simulink model "ClosedLoopControl"  (R2016b)
settings: Solver=FixedStepDiscrete  StartTime=0.0  StopTime=Inf  FixedStep=sCoreParams.core.stepPeriod  RelTol=1e-3  EnableMultiTasking=on
undefined symbols (not defined in the file): fdesignblkfcn, gcbh, High, sCoreParams, sCoreParams_decoders_chanceDetector_randStimEventsPerSec, sCoreParams_decoders_txDetector_channel1, sCoreParams_decoders_txDetector_channel2, sCoreParams_decoders_txDetector_detectChannelInds, sCoreParams_decoders_txDetector_nChannels, sCoreParams_Features_Baseline_initialThresholdValue, sCoreParams_Features_Baseline_weightPreviousThreshold, sCoreParams_Features_Data_SmoothWindowsDurationSamples, sCoreParams_stimulator_stimAfterDelaySteps
libraries: dsparch4 x20, dspstat3 x19, dspspect3 x6, dspfdesign x2, dspindex x2, dspswit3 x1
(part 6 of 6)

== system ClosedLoopControl/FilterBanks/Variant FILTER 2000/65-200Hz HighGammaRipple FIR ==
  EEGData : Inport
  Generated Filter Block : DiscreteFir  Tag=BlockMethodSubSystem  Coefficients=[0.043674950645707943 -0.010510801076776438 -0.0092198604406533054 -0.0078072197440863019 -0.0061576291109547441 -0.0043314949479796505 -0.0026149837714866844 -0.0014281197315007387 -0.0011887830977032846 -0.0020631394359844836 -0.0038906609829976006 -0.006134979543899413 -0.0080743521554436769 -0.0090186910392010006 -0.0085928718984132329 -0.0068824719973744029 -0.0044344002598706734 -0.0020632098371482117 -0.00054620058864337216 -0.00031706926836648172 -0.0012806039208504247 -0.0028303540771732584 -0.0040768356042938676 -0.004193132697654047 -0.0027660676413756961 1.9003693936618729e-05 0.0034067519279456487 0.0063472526354222602 0.0078958974614977504 0.0075793823939889725 0.0056281036442865778 0.0028514070097576216 0.00042987516134896416 -0.00071303834093239911 1.1697363323633972e-05 0.0020369008242335485 0.0045707172575817877 0.0063400232285504843 0.006152335767163339 0.003695198751154251 -0.00054923784249524951 -0.0052930021300986009 -0.009082894815013105 -0.010679189468049901 -0.009713948692912408 -0.0067468353855187129 -0.0031802128714443988 -0.00063228620545409213 -0.00035139072256231481 -0.0026086409852362456 -0.0065830274486462651 -0.010571501918713583 -0.012689614383126465 -0.011577477565379819 -0.0070576745373317736 -0.00022999532853976319 0.0068154951113979841 0.011843234875324286 0.013289460151243533 0.011001391875699177 0.0063095176650106582 0.0016313362199767314 -0.00052119400123590027 0.0014569178651438908 0.0074726777669980133 0.015628713969671838 0.022826703629726497 0.025893486581749524 0.022907578453487763 0.014019972540609493 0.0016645482174998925 -0.010167457554019462 -0.017562158381230882 -0.0180477323755667 -0.01194498020464765 -0.0024264873025872094 0.0052207045747070255 0.0056493327084122186 -0.0045373885153166225 -0.025015012812241458 -0.051246002878708945 -0.075349015080128312 -0.088355355358379697 -0.083035398155685114 -0.056553784398185536 -0.011862247095400281 0.042515847778265718 0.094576601537287724 0.13197925194672577 0.14558091380700244 0.13197925194672577 0.094576601537287724 0.042515847778265718 -0.011862247095400281 -0.056553784398185536 -0.083035398155685114 -0.088355355358379697 -0.075349015080128312 -0.051246002878708945 -0.025015012812241458 -0.0045373885153166225 0.0056493327084122186 0.0052207045747070255 -0.0024264873025872094 -0.01194498020464765 -0.0180477323755667 -0.017562158381230882 -0.010167457554019462 0.0016645482174998925 0.014019972540609493 0.022907578453487763 0.025893486581749524 0.022826703629726497 0.015628713969671838 0.0074726777669980133 0.0014569178651438908 -0.00052119400123590027 0.0016313362199767314 0.0063095176650106582 0.011001391875699177 0.013289460151243533 0.011843234875324286 0.0068154951113979841 -0.00022999532853976319 -0.0070576745373317736 -0.011577477565379819 -0.012689614383126465 -0.010571501918713583 -0.0065830274486462651 -0.0026086409852362456 -0.00035139072256231481 -0.00063228620545409213 -0.0031802128714443988 -0.0067468353855187129 -0.009713948692912408 -0.010679189468049901 -0.009082894815013105 -0.0052930021300986009 -0.00054923784249524951 0.003695198751154251 0.006152335767163339 0.0063400232285504843 0.0045707172575817877 0.0020369008242335485 1.1697363323633972e-05 -0.00071303834093239911 0.00042987516134896416 0.0028514070097576216 0.0056281036442865778 0.0075793823939889725 0.0078958974614977504 0.0063472526354222602 0.0034067519279456487 1.9003693936618729e-05 -0.0027660676413756961 -0.004193132697654047 -0.0040768356042938676 -0.0028303540771732584 -0.0012806039208504247 -0.00031706926836648172 -0.00054620058864337216 -0.0020632098371482117 -0.0044344002598706734 -0.0068824719973744029 -0.0085928718984132329 -0.0090186910392010006 -0.0080743521554436769 -0.006134979543899413 -0.0038906609829976006 -0.0020631394359844836 -0.0011887830977032846 -0.0014281197315007387 -0.0026149837714866844 -0.0043314949479796505 -0.0061576291109547441 -0.0078072197440863019 -0.0092198604406533054 -0.010510801076776438 0.043674950645707943]  InputProcessing=Columns as channels (frame based)
  filteredData : Outport
  wires:
  EEGData/1 -> Generated Filter Block/1
  Generated Filter Block/1 -> filteredData/1

== system ClosedLoopControl/FilterBanks/Variant FILTER 2000/65-200Hz HighGammaRipple IIR ==
  EEGData : Inport
  Generated Filter Block : dsparch4/Biquad Filter  Tag=BlockMethodSubSystem  IIRFiltStruct=Direct form II  CoeffSource=Specify via dialog  BiQuadCoeffs=[0.67667743659925317 0 -0.67667743659925317 1 -1.791106372362715 0.84351743161553339;0.20837637004489881 0 -0.20837637004489881 1 -1.4769568640840638 0.82858480682365565;0.21913950715217931 0 -0.21913950715217931 1 -1.3946221573759421 0.62632638513627259;0.13404107548876229 0 -0.13404107548876229 1 -1.4634270346154397 0.61227676045926838;0.22926259000998553 0 -0.22926259000998553 1 -1.4248965089945402 0.73918023284028478;0.1662719018063869 0 -0.1662719018063869 1 -1.6043511746437273 0.69199629969542564;0.071396379929834025 0 -0.071396379929834025 1 -1.9317179351880835 0.97744998664625005;0.26148164315809597 0 -0.26148164315809597 1 -1.5540993535626753 0.93822820155749087;0.25565951467668901 0 -0.25565951467668901 1 -1.7364105251114004 0.79566729073556186;0.21891419381257862 0 -0.21891419381257862 1 -1.6744829666918539 0.74473352537242943;0.16735244352374978 0 -0.16735244352374978 1 -1.4166978728907922 0.60600668409114;0.2415146980022162 0 -0.2415146980022162 1 -1.3974831127623975 0.6713282499392339;0.26540418737962024 0 -0.26540418737962024 1 -1.5300311665420243 0.64388417032152689;0.10300734712666591 0 -0.10300734712666591 1 -1.8869858981947756 0.93319650449939318;2 0 -2 1 -1.8406560359772179 0.88897180839051049]  a0Flag=Warning  IC=0  ICnum=0  ICden=0  InputProcessing=Columns as channels (frame based)  denAccumFracLength=30  denProdOutputFracLength=30  secondMemoryFracLength=15  roundingMode=Floor  overflowMode=off  ScaleValues=[0.034709882337591945;1;1;1;1;1;1;1;1;1;1;1;1;1;1;1.0919362488362816]  optimizeScaleValues=off  ScaleValueMode=Specify via input port (g)  scaleValueFracLength=14  FilterSource=Specify via dialog  FilterObject=BQF
  filteredData : Outport
  wires:
  EEGData/1 -> Generated Filter Block/1
  Generated Filter Block/1 -> filteredData/1

== system ClosedLoopControl/FilterBanks/Variant FILTER 2000/8-15Hz Alpha FIR ==
  EEGData : Inport
  Generated Filter Block : DiscreteFir  Tag=BlockMethodSubSystem  Coefficients=[1.1166843982614926e-06 -5.1505963497875887e-06 -1.2812602333555129e-05 -2.1871054990882468e-05 -3.2323373818540652e-05 -4.4162634838047868e-05 -5.7377540676991869e-05 -7.195240245586386e-05 -8.7867133639842035e-05 -0.00010509725598372113 -0.00012361391766630315 -0.00014338392367813367 -0.000164369778493665 -0.00018652974102566303 -0.00020981789182618625 -0.0002341842124648283 -0.0002595746769810637 -0.00028593135527383055 -0.00031319252825774447 -0.00034129281458180586 -0.00037016330867327857 -0.00039973172983648352 -0.00042992258210380332 -0.00046065732450443646 -0.00049185455138502153 -0.00052343018238589314 -0.000555297661646971 -0.0005873681657885076 -0.00061955082018408858 -0.00065175292301663287 -0.00068388017658249981 -0.00071583692528446631 -0.00074752639973140443 -0.00077885096634068161 -0.00080971238181931681 -0.00084001205188102607 -0.00086965129353934944 -0.00089853160030159028 -0.0009265549095744043 -0.00095362387157998788 -0.00097964211907159478 -0.0010045145371285577 -0.0010281475323047058 -0.0010504493003992363 -0.0010713300921165658 -0.0010907024758808866 -0.0011084815970723843 -0.0011245854329553625 -0.00113893504257369 -0.0011514548108961891 -0.001162072686503848 -0.0011707204121218695 -0.0011773337473127315 -0.0011818526826615754 -0.0011842216448022078 -0.0011843896916509528 -0.0011823106972363748 -0.0011779435255354414 -0.00117125219275111 -0.0011622060174923557 -0.0011507797583454361 -0.001136953738354511 -0.0011207139559606311 -0.0011020521819804436 -0.0010809660422397137 -0.001057459085511797 -0.0010315408364474827 -0.0010032268332200427 -0.00097253864964778316 -0.00093950390159584351 -0.00090415623749921738 -0.00086653531289007147 -0.00082668674885407638 -0.00078466207438273922 -0.00074051865263137029 -0.00069431959113537079 -0.0006461336360806941 -0.00059603505076769926 -0.00054410347845094465 -0.00049042378978056769 -0.0004350859151140158 -0.00037818466200922462 -0.0003198195182527428 -0.00026009444081761201 -0.00019911763118664756 -0.00013700129751690498 -7.3861404160011573e-05 -9.8174090911267554e-06 5.5008010163797022e-05 0.00012048924147724876 0.00018649803328639865 0.00025290379928409514 0.00031957393191114501 0.00038637412389685354 0.00045316869706702476 0.00051982093761261162 0.00058619343698820684 0.00065214843758748075 0.00071754818232275524 0.00078225526721801533 0.00084613299610908864 0.00090904573653135254 0.00097085927586427958 0.0010314411767934721 0.0010906611311446244 0.0011483913111399052 0.0012045067171260633 0.0012588855208245753 0.0013114094031579228 0.0013619638857121615 0.0014104386549047448 0.0014567278779377545 0.0015007305096304167 0.0015423505892410412 0.0015814975264072709 0.001618086375354588 0.0016520380965466808 0.0016832798049771526 0.0017117450043303123 0.0017373738062692796 0.0017601131341423238 0.0017799169104332252 0.0017967462273182613 0.0018105694997313348 0.0018213626003794627 0.0018291089761933916 0.0018337997457423454 0.0018354337771877447 0.0018340177463980255 0.0018295661748954481 0.0018221014473556757 0.0018116538084320456 0.0017982613387285684 0.0017819699097986867 0.0017628331181006056 0.0017409121978943678 0.0017162759131207782 0.0016890004283574528 0.0016591691590027344 0.0016268726008937253 0.001592208139620101 0.0015552798398505627 0.0015161982150436648 0.0014750799779690521 0.0014320477725188181 0.0013872298873415828 0.0013407599518838245 0.0012927766154738488 0.001243423210133381 0.0011928473978500983 0.0011412008030911467 0.0010886386313827949 0.0010353192748249133 0.00098140390545031655 0.0009270560573785804 0.00087244119875139019 0.00081772629447154682 0.00076307936080061199 0.00070866901290059193 0.00065466400643282975 0.00060123277435255879 0.00054854296006001896 0.00049676094808876381 0.00044605139352870261 0.00039657675139517979 0.00034849680716653192 0.0003019682097202846 0.00025714400790310016 0.00021417319197122785 0.00017320024113676101 0.00013436467845048239 9.7800634244212941e-05 6.3636419344704006e-05 3.1994109256920648e-05 ...(+13836 chars)]  InputProcessing=Columns as channels (frame based)
  filteredData : Outport
  wires:
  EEGData/1 -> Generated Filter Block/1
  Generated Filter Block/1 -> filteredData/1

== system ClosedLoopControl/FilterBanks/Variant FILTER 2000/8-15Hz Alpha IIR ==
  EEGData : Inport
  Generated Filter Block : dsparch4/Biquad Filter  Tag=BlockMethodSubSystem  IIRFiltStruct=Direct form II  CoeffSource=Specify via dialog  BiQuadCoeffs=[0.015868678952687381 0 -0.015868678952687381 1 -1.9863057355894018 0.98849302872752898;0.012908102499795312 0 -0.012908102499795312 1 -1.9847266874502132 0.98549663747335259;0.012163285852299357 0 -0.012163285852299357 1 -1.9771841889355546 0.9782509221793142;0.0036350465229467144 0 -0.0036350465229467144 1 -1.9761530939602661 0.97794142504950965;0.013108401993006964 0 -0.013108401993006964 1 -1.9973187714207226 0.9979309482534352;0.0090946861417868265 0 -0.0090946861417868265 1 -1.9937226181401737 0.99600642262399586;0.016480983831500946 0 -0.016480983831500946 1 -1.9802455114003683 0.98226074636179173;0.015172775510067973 0 -0.015172775510067973 1 -1.9806785345565951 0.98157317499958641;0.013635778665057739 0 -0.013635778665057739 1 -1.9748579961420645 0.97614296928413746;0.016343732373669716 0 -0.016343732373669716 1 -1.9743690299553807 0.97590353767478455;0.0091422519026776641 0 -0.0091422519026776641 1 -1.9931527192109855 0.99378819123385109;2 0 -2 1 -1.9889418875963765 0.98962803867229587]  a0Flag=Warning  IC=0  ICnum=0  ICden=0  InputProcessing=Columns as channels (frame based)  denAccumFracLength=30  denProdOutputFracLength=30  secondMemoryFracLength=15  roundingMode=Floor  overflowMode=off  ScaleValues=[0.00053568024160976873;1;1;1;1;1;1;1;1;1;1;1;9.5315398355264662]  optimizeScaleValues=off  ScaleValueMode=Specify via input port (g)  scaleValueFracLength=14  FilterSource=Specify via dialog  FilterObject=BQF
  filteredData : Outport
  wires:
  EEGData/1 -> Generated Filter Block/1
  Generated Filter Block/1 -> filteredData/1

== system ClosedLoopControl/FilterBanks/Variant FILTER 2000/80-200Hz HFORipple FIR ==
  EEGData : Inport
  Generated Filter Block : DiscreteFir  Tag=BlockMethodSubSystem  Coefficients=[-0.029929468383316192 0.027584903344857116 0.006558984880081789 -0.0071603267655065833 -0.013247180355273648 -0.013135920645701411 -0.0090343519140387157 -0.0032754151064268641 0.0022272516299482945 0.0061526392461596219 0.0079390912269469774 0.0076686887032404866 0.0060227556600073798 0.0039349955485136062 0.002396304305429954 0.0020527359637715833 0.0031029488412524647 0.0051247167458305515 0.0073477544104056103 0.0087957682525686351 0.0088043284423398316 0.00710059570242208 0.0041318613604908808 0.00067350576530127854 -0.0021332528816080248 -0.0036147405910317496 -0.0034016416976209995 -0.001904243925895048 -9.8116221945575288e-05 0.0011838227951950983 0.0010052402801807789 -0.00069375398602379568 -0.0033161108088197999 -0.0058093921651041838 -0.0070688296122434977 -0.0062279411320784531 -0.0032465358048272691 0.0011033746367409905 0.0054903794295953143 0.0085941785365106216 0.0095047981352248956 0.0081292793472463598 0.005237259579484288 0.0022388728520793405 0.00053886046527349546 0.00096339401712913775 0.0033698853216399469 0.006695473988653354 0.0093294470183197739 0.009730061973901652 0.0070986567584101143 0.0017181031971334401 -0.0049383095140956221 -0.010887765954854724 -0.014221289453944019 -0.013976819805220315 -0.010530893082807774 -0.0054287582554014349 -0.00088011910410184385 0.0011679539587099719 -0.00014547643883787431 -0.0041760754011632081 -0.008944366661674398 -0.011801424674010449 -0.010562162379392094 -0.0044555321547889229 0.0053958544645990661 0.016263138140394436 0.024694650965907963 0.027841496662202841 0.024596298085779726 0.016203929024829047 0.0058734470287940752 -0.0023244041555813555 -0.0050790680728182019 -0.0012630785826390906 0.0072633206754821183 0.016070445540513408 0.019596048919655211 0.013222985157710941 -0.0046438574372398012 -0.031492102130720984 -0.060763349522214613 -0.083541115124259574 -0.09120184118086383 -0.078307752643135484 -0.04470543854444764 0.0038254224665319886 0.056784017626830177 0.10164096275331343 0.12730747905853101 0.12730747905853101 0.10164096275331343 0.056784017626830177 0.0038254224665319886 -0.04470543854444764 -0.078307752643135484 -0.09120184118086383 -0.083541115124259574 -0.060763349522214613 -0.031492102130720984 -0.0046438574372398012 0.013222985157710941 0.019596048919655211 0.016070445540513408 0.0072633206754821183 -0.0012630785826390906 -0.0050790680728182019 -0.0023244041555813555 0.0058734470287940752 0.016203929024829047 0.024596298085779726 0.027841496662202841 0.024694650965907963 0.016263138140394436 0.0053958544645990661 -0.0044555321547889229 -0.010562162379392094 -0.011801424674010449 -0.008944366661674398 -0.0041760754011632081 -0.00014547643883787431 0.0011679539587099719 -0.00088011910410184385 -0.0054287582554014349 -0.010530893082807774 -0.013976819805220315 -0.014221289453944019 -0.010887765954854724 -0.0049383095140956221 0.0017181031971334401 0.0070986567584101143 0.009730061973901652 0.0093294470183197739 0.006695473988653354 0.0033698853216399469 0.00096339401712913775 0.00053886046527349546 0.0022388728520793405 0.005237259579484288 0.0081292793472463598 0.0095047981352248956 0.0085941785365106216 0.0054903794295953143 0.0011033746367409905 -0.0032465358048272691 -0.0062279411320784531 -0.0070688296122434977 -0.0058093921651041838 -0.0033161108088197999 -0.00069375398602379568 0.0010052402801807789 0.0011838227951950983 -9.8116221945575288e-05 -0.001904243925895048 -0.0034016416976209995 -0.0036147405910317496 -0.0021332528816080248 0.00067350576530127854 0.0041318613604908808 0.00710059570242208 0.0088043284423398316 0.0087957682525686351 0.0073477544104056103 0.0051247167458305515 0.0031029488412524647 0.0020527359637715833 0.002396304305429954 0.0039349955485136062 0.0060227556600073798 0.0076686887032404866 0.0079390912269469774 0.0061526392461596219 0.0022272516299482945 -0.0032754151064268641 -0.0090343519140387157 -0.013135920645701411 -0.013247180355273648 -0.0071603267655065833 0.006558984880081789 0.027584903344857116 -0.029929468383316192]  InputProcessing=Columns as channels (frame based)
  filteredData : Outport
  wires:
  EEGData/1 -> Generated Filter Block/1
  Generated Filter Block/1 -> filteredData/1

== system ClosedLoopControl/FilterBanks/Variant FILTER 2000/80-200Hz HFORipple IIR ==
  EEGData : Inport
  Generated Filter Block : dsparch4/Biquad Filter  Tag=BlockMethodSubSystem  IIRFiltStruct=Direct form II  CoeffSource=Specify via dialog  BiQuadCoeffs=[0.24712034122740287 0 -0.24712034122740287 1 -1.4983491296398279 0.85456538800842674;0.16863512188048954 0 -0.16863512188048954 1 -1.7857549325984627 0.8524261725854152;0.21026427858880101 0 -0.21026427858880101 1 -1.4191660026684048 0.67094248798924361;0.19677748510054191 0 -0.19677748510054191 1 -1.5090368136491961 0.65492200060340777;0.14251414265837331 0 -0.14251414265837331 1 -1.6829941372716386 0.76639535035267592;0.029415958678099235 0 -0.029415958678099235 1 -1.6253971757107712 0.72350968856028086;0.61614731970082015 0 -0.61614731970082015 1 -1.9183031603651139 0.97839278350900338;0.10675070099208174 0 -0.10675070099208174 1 -1.5643791756503553 0.94815577400739715;0.26295811976493666 0 -0.26295811976493666 1 -1.7364311148941871 0.80976110546851021;0.1951049824225832 0 -0.1951049824225832 1 -1.4522317691443489 0.77624533936164397;0.21097875272858438 0 -0.21097875272858438 1 -1.4316675822483291 0.64614036167249;0.14511741935080547 0 -0.14511741935080547 1 -1.4625208221331381 0.64100286620384839;0.22920714130008057 0 -0.22920714130008057 1 -1.4259153430128997 0.7146613453186289;0.25503819054827076 0 -0.25503819054827076 1 -1.5656754220651468 0.68443780762870654;0.11170944942250573 0 -0.11170944942250573 1 -1.8756699106981227 0.93612021907193865;1.926779228382183 0 -1.926779228382183 1 -1.8318227982981279 0.89437772655414227]  a0Flag=Warning  IC=0  ICnum=0  ICden=0  InputProcessing=Columns as channels (frame based)  denAccumFracLength=30  denProdOutputFracLength=30  secondMemoryFracLength=15  roundingMode=Floor  overflowMode=off  ScaleValues=[0.08520268411340283;1;1;1;1;1;1;1;1;1;1;1;1;1;1;1;1]  optimizeScaleValues=off  ScaleValueMode=Specify via input port (g)  scaleValueFracLength=14  FilterSource=Specify via dialog  FilterObject=BQF
  filteredData : Outport
  wires:
  EEGData/1 -> Generated Filter Block/1
  Generated Filter Block/1 -> filteredData/1

== system ClosedLoopControl/FilterBanks/Variant FILTER 2000/AllBand ==
  EEGData : Inport
  filteredData : Outport
  wires:
  EEGData/1 -> filteredData/1

== system ClosedLoopControl/FilterBanks/Variant FILTER 2000/VariableFreq FIR ==
  EEGData : Inport
  Discrete FIR Filter : DiscreteFir  FilterStructure=Direct form symmetric  Coefficients=sCoreParams.filter.Hd.Numerator
  filteredData : Outport
  wires:
  Discrete FIR Filter/1 -> filteredData/1
  EEGData/1 -> Discrete FIR Filter/1

== system ClosedLoopControl/Variant THRESHOLDS/WeightedBandPowerInTime/Compute Smooth Power as ^2 ==
  In1 : Inport
  Trigger : TriggerPort  VariantControl=Variant  PortDimensions=1
  Buffer1 : Buffer  N=sCoreParams.Features.Baseline.SmoothWindowsDurationSamples  V=sCoreParams.Features.Baseline.SmoothWindowsDurationSamples-1  TreatMby1Signals=One channel
  Frame Conversion1 : FrameConversion  InheritSamplingMode=off  OutFrame=Sample-based
  Mean1 : dspstat3/Mean  run=off  reset_popup=None  InputProcessing=Columns as channels (frame based)  directionMode=Each column  dimension=1  roiEnable=off  roiType=Rectangles  roiPortion=Entire ROI  roiOutput=Individual statistics for each ROI  roiFlag=off  outputDataTypeStr=Inherit: Same as accumulator  outputLastDataTypeStr=Inherit: Same as accumulator  outputMin=[]  outputMax=[]  roundingMode=Floor  overflowMode=off
  Mean2 : dspstat3/Mean  run=off  reset_popup=None  InputProcessing=Columns as channels (frame based)  directionMode=Each column  dimension=1  roiEnable=off  roiType=Rectangles  roiPortion=Entire ROI  roiOutput=Individual statistics for each ROI  roiFlag=off  outputDataTypeStr=Inherit: Same as accumulator  outputLastDataTypeStr=Inherit: Same as accumulator  outputMin=[]  outputMax=[]  roundingMode=Floor  overflowMode=off
  Product : Product
  Out1 : Outport
  wires:
  Mean1/1 -> Frame Conversion1/1
  In1/1 -> Product/1, Product/2
  Buffer1/1 -> Mean1/1
  Product/1 -> Mean2/1
  Mean2/1 -> Buffer1/1
  Frame Conversion1/1 -> Out1/1

== system ClosedLoopControl/Variant THRESHOLDS/WeightedCoherence/Compute Coherence ==
  In2 : Inport
  Trigger : TriggerPort  VariantControl=Variant
  Constant : Constant  Value=sCoreParams.core.samplingRate
  Frame Conversion1 : FrameConversion  InheritSamplingMode=off  OutFrame=Sample-based
  detectableChannels : Constant  Value=sCoreParams_decoders_txDetector_detectChannelInds
  highFreq : Constant  Value=sCoreParams.Features.Coherence.highFreq
  lowFreq : Constant  Value=sCoreParams.Features.Coherence.lowFreq
  runAvCoherence : MATLAB Function  TreatAsAtomicUnit=on
  Out2 : Outport  InitialOutput=sCoreParams.Features.Baseline.initialThresholdValue
  wires:
  runAvCoherence/1(coherenceValue) -> Frame Conversion1/1  "coherencePerChannel"
  Constant/1 -> runAvCoherence/4(Fs)
  lowFreq/1 -> runAvCoherence/2(lowFreq)
  highFreq/1 -> runAvCoherence/3(highFreq)
  Frame Conversion1/1 -> Out2/1
  In2/1 -> runAvCoherence/1(filteredData)
  detectableChannels/1 -> runAvCoherence/5(detectChannelInds)

== system ClosedLoopControl/Variant THRESHOLDS/WeightedCorrelation/Compute Correlation ==
  In1 : Inport
  Trigger : TriggerPort  VariantControl=Variant  PortDimensions=1
  Frame Conversion1 : FrameConversion  InheritSamplingMode=off  OutFrame=Sample-based
  xCorrCoef : MATLAB Function  TreatAsAtomicUnit=on
  Out1 : Outport
  wires:
  In1/1 -> xCorrCoef/1(filteredData)
  xCorrCoef/1(rxy) -> Frame Conversion1/1
  Frame Conversion1/1 -> Out1/1

== system ClosedLoopControl/Variant THRESHOLDS/WeightedVarianceOfPower/Compute Variance of Power ==
  In1 : Inport
  Trigger : TriggerPort  VariantControl=Variant
  Magnitude FFT : dspspect3/Magnitude FFT  mag_or_magsq=Magnitude squared  FFTImplementation=Auto  fftLenInherit=on  fftsize=32  WrapInput=on
  Mean : dspstat3/Mean  run=off  reset_popup=None  InputProcessing=Columns as channels (frame based)  directionMode=Each column  dimension=1  roiEnable=off  roiType=Rectangles  roiPortion=Entire ROI  roiOutput=Individual statistics for each ROI  roiFlag=off  outputDataTypeStr=Inherit: Same as accumulator  outputLastDataTypeStr=Inherit: Same as accumulator  outputMin=[]  outputMax=[]  roundingMode=Floor  overflowMode=off
  Variance : dspstat3/Variance  run=off  reset_popup=None  InputProcessing=Columns as channels (frame based)  directionMode=Each column  dimension=1  roiEnable=off  roiType=Rectangles  roiPortion=Entire ROI  roiOutput=Individual statistics for each ROI  roiFlag=off  roundingMode=Floor  overflowMode=off
  Out1 : Outport
  wires:
  In1/1 -> Magnitude FFT/1
  Magnitude FFT/1 -> Variance/1
  Variance/1 -> Mean/1
  Mean/1 -> Out1/1

== matlab function ClosedLoopControl/Detection/Random (Sham) Detection ==
  data: detectShamBool input; shamEventDetected output; targetShamFrequencySec input; stepPeriod input
function shamEventDetected = RandomDetector(detectShamBool, targetShamFrequencySec, stepPeriod)
%#codegen

if detectShamBool>0 && targetShamFrequencySec>0 %Only stim if detectShamBool SET to 1 and at targetShamFrequencySec is not zero (so it can be turnned off from GUI)
    shamEventDetected = ShamDetector_EML(detectShamBool, targetShamFrequencySec, stepPeriod);
else
    shamEventDetected = false;
end

== matlab function ClosedLoopControl/Variant THRESHOLDS/WeightedCorrelation/Compute Correlation/xCorrCoef ==
  data: filteredData input; rxy output size=sCoreParams.decoders.txDetector.nPairs
function rxy = compCorrelation(filteredData)
%#codegen

[rxy] = compCorrelation_EML(filteredData);

== matlab function ClosedLoopControl/Variant FEATURES/Correlation/xCorrCoef ==
  data: filteredData input; rxy output
function rxy = compCorrelation(filteredData)
%#codegen

[rxy] = compCorrelation_EML(filteredData);

== matlab function ClosedLoopControl/Variant THRESHOLDS/WeightedCoherence/Compute Coherence/runAvCoherence ==
  data: filteredData input; coherenceValue output; lowFreq input; highFreq input; Fs input; detectChannelInds input
function coherenceValue   = runCoherence(filteredData, lowFreq, highFreq, Fs, detectChannelInds)
%#codegen
% Run mscohere in filteredData
% Returns magnitude-square coherence between pairs of channels for the whole time window

[~, avCoherence, coherenceValue, pairChannels] = runCoherence_EML(filteredData, lowFreq, highFreq, Fs, detectChannelInds);
%[sumCoherencePerChannel, avCoherence, coherenceValue] = runCoherenceMultitaper_EML(filteredData, lowFreq, highFreq, nPoints, Fs);
